simulink model "Sim5"  (R2014a)
settings: Solver=ode45  StartTime=0.0  StopTime=10.0  RelTol=1e-3
settings Model: Creator=OCAC  LastModifiedBy=OCAC

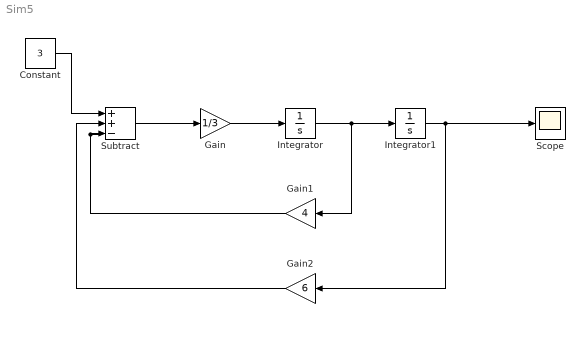
== system Sim5 ==
  Constant : Constant  Value=3
  Gain : Gain  Gain=1/3
  Gain1 : Gain  Gain=4
  Gain2 : Gain  Gain=6
  Integrator : Integrator
  Integrator1 : Integrator
  Scope : Scope
  Subtract : Sum  Inputs=++-
  wires:
  Gain/1 -> Integrator/1
  Constant/1 -> Subtract/1
  Integrator/1 -> Gain1/1, Integrator1/1
  Subtract/1 -> Gain/1
  Integrator1/1 -> Scope/1, Gain2/1
  Gain1/1 -> Subtract/3
  Gain2/1 -> Subtract/2
